simulink model "buck_converter_sic"  (R2025a)
settings: Solver=ode23t  StartTime=0.0  StopTime=0.01  MaxStep=1e-9  RelTol=1e-7
undefined symbols (not defined in the file): Acid, Lead
libraries: spsMeanLib x6, spsSeriesRLCBranchLib x4, spsCurrentMeasurementLib x2, spsMosfetLib x2, spsVoltageMeasurementLib x2, spsBatteryLib x1, spsGroundLib x1, spsPVArrayLib x1, simulink x1, sps_lib x1
settings Model: Creator=Dell  LastModifiedBy=Harish
settings SolverCC: AlgebraicLoopSolver=TrustRegion
settings DebuggingCC: UnconnectedInputMsg=warning  UnconnectedOutputMsg=warning  UnconnectedLineMsg=warning
settings ModelReferenceCC: EnableRefExpFcnMdlSchedulingChecks=on
settings RTWCC: GPUComputeCapability=3.5  DLArmComputeVersion=19.05

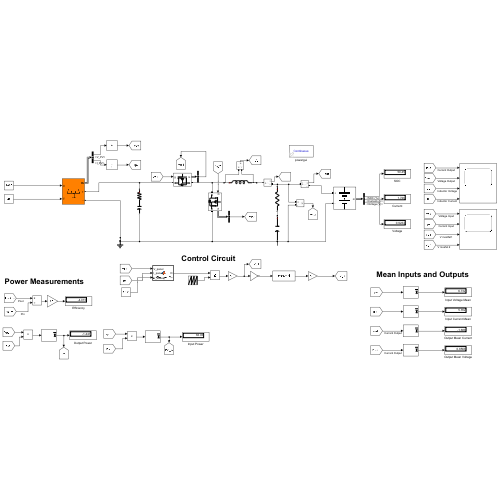
[thumbnail: Simulink's stored preview of the top-level diagram]
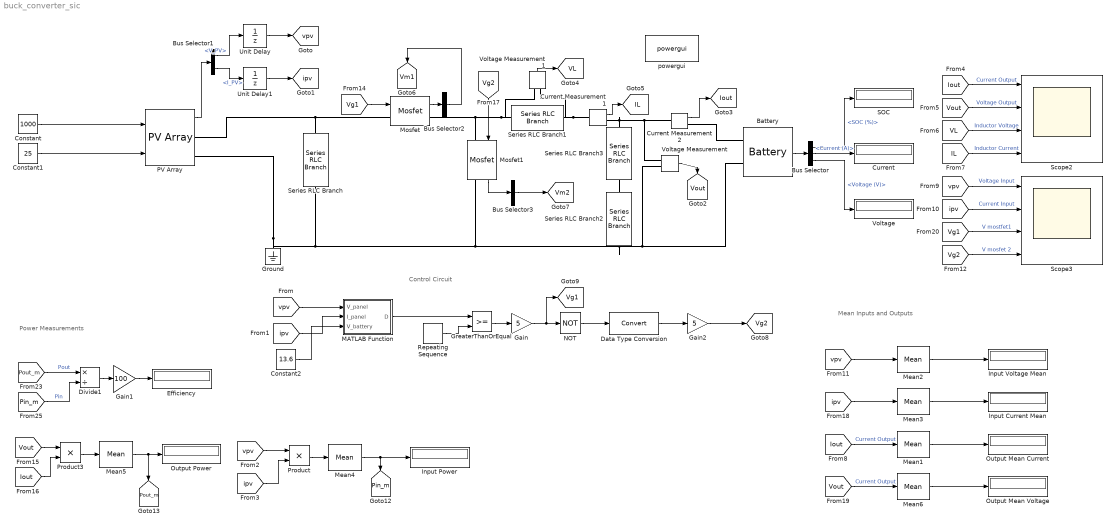
== system buck_converter_sic ==
  note: Mean Inputs and Outputs
  note: Control Circuit
  note: Power Measurements
  Battery : spsBatteryLib/Battery  BatType=Lead-Acid  NomV=14.4  NomQ=7.5  SOC=45  Batt_Tr=1  PresetModel=off  MaxQ=7.8125  MinV=10.8  FullV=15.6789  Dis_rate=1.5  R=0.0192  Normal_OP=2.3271  expZone="[14.6605        0.025]"
      settings: LibrarySourceBlock=electricdrivelib/Extra Sources/Battery
  Bus Selector : BusSelector  OutputSignals=SOC (%),Current (A),Voltage (V)
  Bus Selector1 : BusSelector  OutputSignals=V_PV,I_PV
  Bus Selector2 : BusSelector  OutputSignals=MOSFET voltage  OutputAsBus=on
  Bus Selector3 : BusSelector  OutputSignals=MOSFET voltage  OutputAsBus=on
  Constant : Constant  Value=1000
  Constant1 : Constant  Value=25
  Constant2 : Constant  Value=13.6
  Current : Display
  Current Measurement1 : spsCurrentMeasurementLib/Current Measurement  PhasorSimulation=off  OutputType=Complex  PSBequivalent=0
  Current Measurement2 : spsCurrentMeasurementLib/Current Measurement  PhasorSimulation=off  OutputType=Complex  PSBequivalent=0
  Data Type Conversion : DataTypeConversion  SaturateOnIntegerOverflow=off  RndMeth=Floor
  Divide1 : Product  Inputs=*/
  Efficiency : Display
  Gain : Gain  Gain=5
  Gain1 : Gain  Gain=100
  Gain2 : Gain  Gain=5
  GreaterThanOrEqual : RelationalOperator  OutDataTypeStr=boolean  RndMeth=Simplest  InputSameDT=off
  Ground : spsGroundLib/Ground  LConnTagsString=a
  Input Current Mean : Display
  Input Power : Display
  Input Voltage Mean : Display
  MATLAB Function : MATLAB Function  TreatAsAtomicUnit=on
  Mean{1..6} (6 alike) : spsMeanLib/Mean  Freq=50e3  Vinit=0  Ts=0
  Mosfet : spsMosfetLib/Mosfet  Ron=20e-3  Lon=0  Rd=0.0028  Vfd=0  IC=0  Rs=1e5  Cs=inf  Measurements=on
  Mosfet1 : spsMosfetLib/Mosfet  Ron=20e-3  Lon=0  Rd=0.0028  Vfd=0  IC=0  Rs=1e5  Cs=inf  Measurements=on
  NOT : Logic  Operator=NOT  IconShape=distinctive  AllPortsSameDT=off
  Output Mean Current : Display
  Output Mean Voltage : Display
  Output Power : Display
  PV Array : spsPVArrayLib/PV Array  Npar=1  Nser=1  PlotType=array @ 1000 W/m2 & specified temperatures  S_vec="[ 1000  500  100 ]"  Temp_C_vec="[ 45 25  ]"  ModuleName=Aavid Thermalloy ASMP-180M  PlotWhenSelected=off  Pm=179.914  Ncell=72  Voc=44.2  Isc=5.36  Vm=36.2  Im=4.97  beta_Voc_pc=-0.38595  alpha_Isc_pc=0.043601  beta_Voc=-0.17059  alpha_Isc=0.002337  IL=5.3889  I0=4.2051e-10  nI=1.0281  Rsh=253.1375  Rs=0.47952  RobustModel=off  RobustCellTemperature=313.3991  BAL=on  Tc=1e-6  Tfilter=5e-5
  Product : Product
  Product3 : Product
  Repeating Sequence : simulink/Sources/Repeating Sequence  rep_seq_t=[0 1/50e3]  rep_seq_y=[0 1]
  SOC : Display
  Scope2 : Scope  NumInputPorts=4
      settings: ActiveDisplayYMinimum=-1.8085601937431193  ActiveDisplayYMaximum=0.20095113263812431  DataLoggingVariableName=ScopeData2
  Scope3 : Scope  NumInputPorts=4
      settings: ActiveDisplayYMinimum=5.0869213004535183  ActiveDisplayYMaximum=6.1785313925593979
  Series RLC Branch : spsSeriesRLCBranchLib/Series RLC Branch  LConnTagsString=__new0  RConnTagsString=__new0  BranchType=RC  Resistance=0.01  Inductance=1e-3  SetiL0=off  InitialCurrent=0  Capacitance=100e-6  Setx0=off  InitialVoltage=0  Measurements=None
  Series RLC Branch1 : spsSeriesRLCBranchLib/Series RLC Branch  LConnTagsString=__new0  RConnTagsString=__new0  BranchType=L  Resistance=1  Inductance=150e-6  SetiL0=off  InitialCurrent=0  Capacitance=1e-6  Setx0=off  InitialVoltage=0  Measurements=None
  Series RLC Branch2 : spsSeriesRLCBranchLib/Series RLC Branch  LConnTagsString=__new0  RConnTagsString=__new0  BranchType=C  Resistance=0.1  Inductance=1e-3  SetiL0=off  InitialCurrent=0  Capacitance=220e-6  Setx0=off  InitialVoltage=0  Measurements=None
  Series RLC Branch3 : spsSeriesRLCBranchLib/Series RLC Branch  LConnTagsString=__new0  RConnTagsString=__new0  BranchType=R  Resistance=0.01  Inductance=1e-3  SetiL0=off  InitialCurrent=0  Capacitance=220.6e-6  Setx0=off  InitialVoltage=0  Measurements=None
  Unit Delay : UnitDelay  SampleTime=1e-9  HasFrameUpgradeWarning=on
  Unit Delay1 : UnitDelay  SampleTime=1e-9  HasFrameUpgradeWarning=on
  Voltage : Display
  Voltage Measurement : spsVoltageMeasurementLib/Voltage Measurement  PhasorSimulation=off  OutputType=Complex  PSBequivalent=0
  Voltage Measurement1 : spsVoltageMeasurementLib/Voltage Measurement  PhasorSimulation=off  OutputType=Complex  PSBequivalent=0
  powergui : sps_lib/powergui  Priority=1  SimulationMode=Continuous  SampleTime=1e-7  frequency=60  Iterations=50  frequencyindice=0  Pbase=100e6  ErrMax=1e-4  UnitsV=kV  UnitsW=MW  buscounter=0  FunctionMessages=off  echomessages=off  EnableUseOfTLC=off  CurrentSourceSwitches=off  DisableSnubberDevices=off  DisableRonSwitches=off  DisableVfSwitches=off  DisplayEquations=off  AutomaticDiscreteSolvers=off  SolverType=Tustin/Backward Euler (TBE)  Interpol=off  ExternalGateDelay=off  methode=off  Ts=100  x0status=blocks  SPID=on  SwTol=0  HookPort=off  NonlinearTolerance=1e-4  nMaxIteration=100  ContinueOnMaxIteration=off  RestoreLinks=warning  ResistiveCurrentMeasurement=off  Frange=[0:2:500]  Ylog=off  Xlog=on  ShowGrid=off  save=off  variable=ZData  structure=0  ZoomFFT=off  StartTime=0.0  cycles=1  DisplayStyle=1  fundamental=60  FreqAxis=off  MaxFrequency=1000  frequencyindicesteady=1  RmsSteady=1  display=off
  tag scope: IL=global, Iout=global, Pin_m=global, Pout_m=global, VL=global, Vg1=global, Vg2=global, Vm1=global, Vm2=global, Vout=global, ipv=global, vpv=global
  wires:
  Constant1/1 -> PV Array/2
  Battery/1 -> Bus Selector/1
  Bus Selector/1 -> SOC/1  "<SOC (%)>"
  Bus Selector/3 -> Voltage/1  "<Voltage (V)>"
  Bus Selector/2 -> Current/1  "<Current (A)>"
  PV Array/1 -> Bus Selector1/1
  Bus Selector1/1 -> Unit Delay/1  "<V_PV>"
  Bus Selector1/2 -> Unit Delay1/1  "<I_PV>"
  Unit Delay/1 -> [vpv]
  Unit Delay1/1 -> [ipv]
  MATLAB Function/1(D) -> GreaterThanOrEqual/1
  Repeating Sequence/1 -> GreaterThanOrEqual/2
  Voltage Measurement/1 -> [Vout]
  Gain1/1 -> Efficiency/1
  Divide1/1 -> Gain1/1
  Product3/1 -> Mean5/1
  [Pin_m] -> Divide1/2  "Pin"
  Mean5/1 -> [Pout_m], Output Power/1
  [Pout_m] -> Divide1/1  "Pout"
  [Iout] -> Product3/2
  [Vout] -> Product3/1
  Product/1 -> Mean4/1
  Mean4/1 -> Input Power/1, [Pin_m]
  [ipv] -> Product/2
  [vpv] -> Product/1
  [Iout] -> Scope2/1  "Current Output"
  [Vout] -> Scope2/2  "Voltage Output"
  Voltage Measurement1/1 -> [VL]
  [VL] -> Scope2/3  "Inductor Voltage"
  Current Measurement1/1 -> [IL]
  [IL] -> Scope2/4  "Inductor Current"
  [Iout] -> Mean1/1  "Current Output"
  Mean1/1 -> Output Mean Current/1
  [vpv] -> Scope3/1  "Voltage Input"
  [ipv] -> Scope3/2  "Current Input"
  [vpv] -> Mean2/1
  Mean2/1 -> Input Voltage Mean/1
  Mosfet/1 -> Bus Selector2/1
  Mosfet1/1 -> Bus Selector3/1
  [Vg1] -> Scope3/3  "V mostfet1"
  Bus Selector2/1 -> [Vm1]
  Bus Selector3/1 -> [Vm2]
  Constant/1 -> PV Array/1
  Mean3/1 -> Input Current Mean/1
  [ipv] -> Mean3/1
  [ipv] -> MATLAB Function/2(I_panel)
  [vpv] -> MATLAB Function/1(V_panel)
  GreaterThanOrEqual/1 -> Gain/1
  [Vg2] -> Scope3/4  "V mosfet 2"
  NOT/1 -> Data Type Conversion/1
  Gain/1 -> [Vg1], NOT/1
  Data Type Conversion/1 -> Gain2/1
  [Vg1] -> Mosfet/1
  [Vg2] -> Mosfet1/1
  Mean6/1 -> Output Mean Voltage/1
  [Vout] -> Mean6/1  "Current Output"
  Gain2/1 -> [Vg2]
  Constant2/1 -> MATLAB Function/3(V_battery)
  Current Measurement2/1 -> [Iout]
  connections:
  Mosfet1/RConn1 -- Series RLC Branch2/RConn1 -- Voltage Measurement/LConn2 -- Battery/LConn2 -- Series RLC Branch/RConn1 -- PV Array/RConn2 -- Ground/LConn1
  Series RLC Branch1/LConn1 -- Voltage Measurement1/LConn1 -- Mosfet1/LConn1 -- Mosfet/RConn1
  Voltage Measurement/LConn1 -- Current Measurement2/LConn1 -- Current Measurement1/RConn1 -- Series RLC Branch3/LConn1
  Voltage Measurement1/LConn2 -- Current Measurement1/LConn1 -- Series RLC Branch1/RConn1
  Mosfet/LConn1 -- PV Array/RConn1 -- Series RLC Branch/LConn1
  Series RLC Branch2/LConn1 -- Series RLC Branch3/RConn1
  Current Measurement2/RConn1 -- Battery/LConn1

== matlab function buck_converter_sic/MATLAB Function ==
  settings: updateMethod=DISCRETE
  data: V_panel input; D output; I_panel input; V_battery input
function D = Battery_Charger_Controller(V_panel, I_panel, V_battery)
    % This function implements a two-stage charger (Bulk and Absorption).
    % It uses MPPT for Bulk, and a stable controller for Absorption.
    
    % Inputs:
    % V_panel:   Current voltage from the solar panel.
    % I_panel:   Current current from the solar panel.
    % V_battery: Current voltage of the battery.
    % Output:
    % D:         The calculated duty cycle (0 to 1) for the buck converter.
    
    %#codegen
    
    % --- 1. Define Charger Parameters & States ---
    ABSORPTION_VOLTAGE = 14.4; % Target voltage for the absorption stage
    FLOAT_VOLTAGE = 13.6;      % Maintenance voltage (state is not reachable)
    
    % State Definitions
    BULK_STATE = 1;
    ABSORPTION_STATE = 2;
    FLOAT_STATE = 3;
    
    % --- Persistent variable to store the current charging stage ---
    persistent charge_stage;
    
    % Initialize the state machine on the first run
    if isempty(charge_stage)
        charge_stage = BULK_STATE; 
    end
    
    % --- 2. State Machine Logic ---
    switch charge_stage
        case BULK_STATE
            % If the battery voltage reaches the absorption level, switch stages.
            if V_battery >= ABSORPTION_VOLTAGE
                charge_stage = ABSORPTION_STATE;
            end
            
        case ABSORPTION_STATE
            % If voltage drops (due to load), it goes back to Bulk.
            % Otherwise, it remains in Absorption mode.
            if V_battery < (ABSORPTION_VOLTAGE - 0.3)
                 charge_stage = BULK_STATE;
            end
            
        case FLOAT_STATE % This state is not reachable in this version
            if V_battery < (FLOAT_VOLTAGE - 0.5)
                charge_stage = BULK_STATE;
            end
    end
    
    % --- 3. Control Action based on State ---
    switch charge_stage
        case BULK_STATE
            % In Bulk stage, our goal is maximum power. Run MPPT.
            D = mppt_p_and_o(V_panel, I_panel);
            
        case ABSORPTION_STATE
            % In Absorption, goal is to hold V_battery at ABSORPTION_VOLTAGE.
            D = voltage_regulator(V_battery, ABSORPTION_VOLTAGE);
            
        case FLOAT_STATE
            % This call is for completeness but the state is unreachable.
            D = voltage_regulator(V_battery, FLOAT_VOLTAGE);
            
        otherwise
            % Safety default
            D = 0; 
    end
end

% --- Helper Function: Perturb & Observe MPPT ---
function D = mppt_p_and_o(V, I)
    % This is a standard Perturb and Observe MPPT algorithm.
    D_MAX = 0.95; D_MIN = 0.05; D_INIT = 0.5; DEL_D = 0.002;
    persistent V_old P_old D_old;
    
    if isempty(V_old)
        V_old = V; P_old = V * I; D_old = D_INIT; D = D_INIT;
        return;
    end
    
    P_new = V * I; dV = V - V_old; dP = P_new - P_old;
    
    if dP > 0
        if dV > 0, D = D_old - DEL_D; else, D = D_old + DEL_D; end
    elseif dP < 0
        if dV > 0, D = D_old + DEL_D; else, D = D_old - DEL_D; end
    else
        D = D_old;
    end
    
    if D > D_MAX, D = D_MAX; elseif D < D_MIN, D = D_MIN; end
    
    D_old = D; V_old = V; P_old = P_new;
end

% --- Helper Function: Voltage Regulator (Stable Version) ---
function D = voltage_regulator(V_actual, V_target)
    % A simple PI-like controller that adjusts the duty cycle incrementally.
    % This version is stable and avoids the voltage collapse issue.
    
    % --- Controller Gain (IMPORTANT: Tune this for your system) ---
    Kp = 0.001; % Start with a SMALL value and increase if needed.
    
    % --- Persistent variable to store the duty cycle ---
    persistent D_persistent;
    
    % Initialize on the first run
    if isempty(D_persistent)
        D_persistent = 0.5; % Start at a 50% duty cycle
    end
    
    % Calculate the error
    error = V_target - V_actual;
    
    % Adjust the duty cycle based on the error
    D_persistent = D_persistent + (error * Kp);
    
    % Clamp the duty cycle to safe limits (0.05 to 0.95)
    if D_persistent > 0.95
        D_persistent = 0.95;
    elseif D_persistent < 0.05
        D_persistent = 0.05;
    end
    
    D = D_persistent;
end
